simulink model "SF5_1_3_db0122_3"  (R2016b)
settings: Solver=FixedStepDiscrete  StartTime=0.0  StopTime=10.0  RelTol=1e-3  EnableMultiTasking=on
PostLoadFcn:
  | % -------------------------------------------------------------------
  | %  Generated by MATLAB on 10-Feb-2017 13:23:05
  | %  MATLAB version: 9.1.0.441655 (R2016b)
  | % -------------------------------------------------------------------
  | 
  | 
  | diffName = Simulink.Signal;
  | diffName.CoderInfo.StorageClass = 'ExportedGlobal';
  | diffName.CoderInfo.Alias = '';
  | diffName.CoderInfo.Alignment = -1;
  | diffName.Description = '';
  | diffName.DataType = 'auto';
  | diffName.Min = [];
  | diffName.Max = [];
  | diffName.DocUnits = '';
  | diffName.Dimensions = -1;
  | diffName.DimensionsMode = 'auto';
  | diffName.Complexity = 'auto';
  | diffName.SampleTime = -1;
  | diffName.InitialValue = '';
  | 
  | myinput = Simulink.Signal;
  | myinput.CoderInfo.StorageClass = 'ExportedGlobal';
  | myinput.CoderInfo.Alias = '';
  | myinput.CoderInfo.Alignment = -1;
  | myinput.Description = '';
  | myinput.DataType = 'auto';
  | myinput.Min = [];
  | myinput.Max = [];
  | myinput.DocUnits = '';
  | myinput.Dimensions = -1;
  | myinput.DimensionsMode = 'auto';
  | myinput.Complexity = 'auto';
  | myinput.SampleTime = -1;
  | myinput.InitialValue = '';
  | 
  | out = Simulink.Signal;
  | out.CoderInfo.StorageClass = 'ExportedGlobal';
  | out.CoderInfo.Alias = '';
  | out.CoderInfo.Alignment = -1;
  | out.Description = '';
  | out.DataType = 'auto';
  | out.Min = [];
  | out.Max = [];
  | out.DocUnits = '';
  | out.Dimensions = -1;
  | out.DimensionsMode = 'auto';
  | out.Complexity = 'auto';
  | out.SampleTime = -1;
  | out.InitialValue = '';
  | 
  | out2 = Simulink.Signal;
  | out2.CoderInfo.StorageClass = 'ExportedGlobal';
  | out2.CoderInfo.Alias = '';
  | out2.CoderInfo.Alignment = -1;
  | out2.Description = '';
  | out2.DataType = 'auto';
  | out2.Min = [];
  | out2.Max = [];
  | out2.DocUnits = '';
  | out2.Dimensions = -1;
  | out2.DimensionsMode = 'auto';
  | out2.Complexity = 'auto';
  | out2.SampleTime = -1;
  | out2.InitialValue = '';
  | 
  | param = Simulink.Parameter;
  | param.Value = [1 2 3 4 5];
  | param.CoderInfo.StorageClass = 'ExportedGlobal';
  | param.CoderInfo.Alias = '';
  | param.CoderInfo.Alignment = -1;
  | param.Description = '';
  | param.DataType = 'auto';
  | param.Min = [];
  | param.Max = [];
  | param.DocUnits = '';
model workspace (MAT data in the model file):
  param = Simulink.Parameter
  param.Value = 4
  param.DataType = 'auto'
  param.Dimensions = [1 1]
settings Model: Creator=amyyang  LastModifiedBy=amyyang
settings DataIOCC: LimitDataPoints=on
settings OptimizationCC: DefaultParameterBehavior=Inlined  LifeSpan=1
settings DebuggingCC: AllowSymbolicDim=off  SFUnexpectedBacktrackingDiag=warning  SFNoUnconditionalDefaultTransitionDiag=warning  SFExecutionAtInitializationDiag=none
settings ModelReferenceCC: PropagateSignalLabelsOutOfModel=off
settings RTWCC: SystemTargetFile=ert.tlc  GenCodeOnly=on  TemplateMakefile=ert_default_tmf  Description=Embedded Coder  GenerateReport=on  IncludeHyperlinkInReport=on  LaunchReport=on  GenerateTraceInfo=on  GenerateTraceReport=on  GenerateTraceReportSl=on  GenerateTraceReportSf=on  GenerateTraceReportEml=on
settings CodeAppCC: IgnoreCustomStorageClasses=off
settings ERTTargetCC: GenerateSampleERTMain=on  InlinedParameterPlacement=NonHierarchical  ERTCustomFileTemplate=example_file_process.tlc  ConvertIfToSwitch=off  SuppressUnreachableDefaultCases=off
settings ConfigComp: CovMetricSettings=dw  CovHtmlReporting=on  CovSaveCumulativeToWorkspaceVar=on  CovSaveSingleToWorkspaceVar=on  CovExternalEMLEnable=off

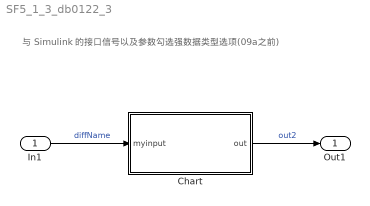
== system SF5_1_3_db0122_3 ==
  note: 与 Simulink 的接口信号以及参数勾选强数据类型选项(09a之前)
  In1 : Inport
  Chart : Stateflow chart  TreatAsAtomicUnit=on
  Out1 : Outport
  wires:
  Chart/1(out) -> Out1/1  "out2"
  In1/1 -> Chart/1(myinput)  "diffName"

== stateflow chart SF5_1_3_db0122_3/Chart ==
  (default) -> (junction 2) : {
      | out = param*myinput;
      | }
  data: out output int32; myinput input int32; param parameter
